simulink model "Virtual_Exhaust_Aftertreatment_Controller_PRT"  (R2016b)
settings: Solver=FixedStepAuto  StartTime=0.0  StopTime=inf  FixedStep=VirtExhATCtrlr.tiSimnTiStep_C  RelTol=1e-3  SampleTimeConstraint=STIndependent  EnableMultiTasking=on
undefined symbols (not defined in the file or in its folder): CAL, SOUIT, T3LIMCL_COEOM_MSK_SY, T3LimCL_stMskEOM1_C, T3LimCL_stMskEOM2_C, T3LimCL_stMskEOM3_C, VirtExhATCtrlr_numHrznSize_CA
libraries: simulink x4
(part 3 of 5)

== system Virtual_Exhaust_Aftertreatment_Controller_PRT/UCatCtrl/SCR_Prediction/Main/UCat NH3 Load Prediction ==
  ATS_tEstUCatAvrg : Inport
  ATS_mflEG : Inport  Port=2
  ATS_facEffUCatAge : Inport  Port=3
  ATS_mflNH3CurrEfc_mgps : Inport  Port=4
  ATS_mflNH3Cnv_mgps : Inport  Port=5
  ATS_stNH3LoadUCatRst : Inport  Port=6
  ATS_mflNH3MetAdapDes_mgps : Inport  Port=7
  ATS_mNH3LoadUCatRst : Inport  Port=8
  ATS_mNH3LoadUCatIni : Inport  Port=9
  Constant1 : Constant  Value=1000  SampleTime=-1
  Constant2 : Constant  Value=0  SampleTime=-1
  Constant6 : Constant  SampleTime=-1
  Constant_1 : Constant  Value=0.02  SampleTime=-1
  Discrete Integrator : Subsystem  mask(Discrete Integrator){}
      mask help:
      | X: Input value
      | Ki: Integral gain
      | Reset: Reset status
      | YReset: Output value during reset
      | Min: Minimum limit of output
      | Max: Maximum limit of output
      | dT : Discrete sample time [sec]
      | Y: Output value
      mask Display:
      | color('blue');
      | fprintf('Discrete\nIntegrator');
      | 
      | color('black');
      | port_label('input', 1, 'X');
      | port_label('input', 2, 'Ki');
      | port_label('input', 3, 'stReset');
      | port_label('input', 4, 'Y0(YReset)');
      | port_label('input', 5, 'Min');
      | port_label('input', 6, 'Max');
      | port_label('input', 7, 'dT');
      | port_label('output', 1, 'Y');
  Divide2 : Product  Inputs=*/
  GOTO_ATS_mflNH3OxiUCatUs_mgps : Subsystem  mask{SIG='ATS_mflNH3OxiUCatUs_mgps'}
      mask prompts: SIG "Log Signal Name"
      mask init: same as Virtual_Exhaust_Aftertreatment_Controller_PRT/UCatCtrl/SCR_Prediction/GOTO_ATS_etaEstNOxCnvUCat
      mask Display: fprintf(SIG);
  Interpolation Using Prelookup : Interpolation_n-D  NumberOfTableDimensions=1  TableSource=Input port  Table=|  ExtrapMethod=Clip  ValidIndexMayReachLast=on
      | [    0.2790    0.2970    0.3080    0.3220    0.3510    0.4240    0.5640    0.6550    0.8190    1.0000    1.0000    1.0000
      |     0.3260    0.3430    0.3540    0.3670    0.3960    0.4660    0.6010    0.6900    0.8440    1.0000    1.0000    1.0000
      |     0.3730    0.3890    0.4000    0.4130    0.4400    0.5080    0.6380    0.7230    0.8680    1.0000    1.0000    1.0000
      |     0.4320    0.4480    0.4580    0.4700    0.4960    0.5600    0.6830    0.7640    0.8970    1.0000    1.0000    1.0000
      |     0.4920    0.5070    0.5160    0.5270    0.5520    0.6120    0.7260    0.8020    0.9220    1.0000    1.0000    1.0000
      |     0.5510    0.5650    0.5730    0.5840    0.6070    0.6620    0.7680    0.8370    0.9410    1.0000    1.0000    1.0000
      |     0.6070    0.6200    0.6280    0.6380    0.6600    0.7130    0.8130    0.8750    0.9580    1.0000    1.0000    1.0000
      |     0.6580    0.6710    0.6790    0.6890    0.7110    0.7630    0.8600    0.9130    0.9730    1.0000    1.0000    1.0000
      |     0.7030    0.7170    0.7250    0.7360    0.7580    0.8130    0.9110    0.9540    0.9900    1.0000    1.0000    1.0000
      |     0.7620    0.7790    0.7900    0.8030    0.8300    0.8980    1.0000    1.0000    1.0000    1.0000    1.0000    1.0000
      |     0.7840    0.7980    0.8060    0.8160    0.8370    0.8910    0.9920    1.0000    1.0000    1.0000    1.0000    1.0000
      |     0.7800    0.8780    0.8820    0.8860    0.8950    0.9180    0.9620    1.0000    1.0000    1.0000    1.0000    1.0000
      | ]
      settings: InputPortMap=u0,u1,p2
  Lookup_n-D_2 : Lookup_n-D  NumberOfTableDimensions=1  BreakpointsForDimension1=[0;0.143;0.286;0.429;0.571;0.714;0.857;1]  Table=[0;0.143;0.286;0.429;0.571;0.714;0.857;1]  ExtrapMethod=Clip  UseLastTableValue=on  RndMeth=Simplest  InputSameDT=on
  Lookup_n-D_3 : Lookup_n-D  BreakpointsForDimension1=[189.96;209.96;229.96;249.96;299.96;349.96;399.96;449.96]  BreakpointsForDimension2=[0 120 200 300 580 700 1040 1500]  Table=[22 22 22 22 22 22 22 22;21.5 21.5 21.5 21.5 21.5 21.5 21.5 21.5;20.7000007629395 20.7000007629395 20.7000007629395 20.7000007629395 20.7000007629395 20.7000007629395 20.7000007629395 20.7000007629395;19.5 19.5 19.5 19.5 19.5 19.5 19.5 19.5;15.5 15.5 15.5 15.5 15.5 15.5 15.5 15.5;11.6999998092651 11.6999998092651 11.6999998092651 11.6999998092651 11.6999998092651 11.6999998092651 11.6999998092651 11.6999998092651;3.79999995231628 3.79999995231628 3.79999995231628 3.79999995231628 3.79999995231628 3.79999995231628 3.79999995231628 3.79999995231628;2.5 2.5 2.5 2.5 2.5 2.5 2.5 2.5]  ExtrapMethod=Clip  UseLastTableValue=on  RndMeth=Simplest  InputSameDT=on
  Lookup_n-D_4 : Lookup_n-D  BreakpointsForDimension1=[189.96;209.96;229.96;249.96;299.96;349.96;399.96;449.96]  BreakpointsForDimension2=[0 120 200 300 580 700 1040 1500]  Table=[29.5009994506836 29.5009994506836 29.5009994506836 29.5009994506836 29.5009994506836 29.5009994506836 29.5009994506836 29.5009994506836;28.2679996490479 28.2679996490479 28.2679996490479 28.2679996490479 28.2679996490479 28.2679996490479 28.2679996490479 28.2679996490479;26.0960006713867 26.0960006713867 26.0960006713867 26.0960006713867 26.0960006713867 26.0960006713867 26.0960006713867 26.0960006713867;22.8250007629395 22.8250007629395 22.8250007629395 22.8250007629395 22.8250007629395 22.8250007629395 22.8250007629395 22.8250007629395;18.5620002746582 18.5620002746582 18.5620002746582 18.5620002746582 18.5620002746582 18.5620002746582 18.5620002746582 18.5620002746582;13.4449996948242 13.4449996948242 13.4449996948242 13.4449996948242 13.4449996948242 13.4449996948242 13.4449996948242 13.4449996948242;4.65299987792969 4.65299987792969 4.65299987792969 4.65299987792969 4.65299987792969 4.65299987792969 4.65299987792969 4.65299987792969;2.49399995803833 2.49399995803833 2.49399995803833 2.49399995803833 2.49399995803833 2.49399995803833 2.49399995803833 2.49399995803833]  ExtrapMethod=Clip  UseLastTableValue=on  RndMeth=Simplest  InputSameDT=on
  Multiport Switch1 : MultiPortSwitch  DataPortOrder=Zero-based contiguous  Inputs=2
  Mux1 : Mux  Inputs=2
  NH3 Oxidation : Subsystem
  Prelookup : PreLookup  BreakpointsData=|  UseLastBreakpoint=on
      | [  0 1.0
      | ]
  Subtract : Sum  Inputs=+-
  Subtract1 : Sum  Inputs=+-
  ATS_mflNH3OxiUCatUs_mgps : Outport
  ATS_mEstNH3LdUCat : Outport  Port=2
  wires:
  ATS_tEstUCatAvrg/1 -> NH3 Oxidation/1(ATS_tEstUCatAvrg), Lookup_n-D_4/1, Lookup_n-D_3/1
  ATS_facEffUCatAge/1 -> NH3 Oxidation/4(ATS_facEffUCatAge), Lookup_n-D_2/1
  ATS_mflEG/1 -> NH3 Oxidation/2(ATS_mflEG), Lookup_n-D_4/2, Lookup_n-D_3/2
  ATS_mflNH3CurrEfc_mgps/1 -> Subtract/1
  Constant1/1 -> Divide2/2
  Divide2/1 -> Discrete Integrator/1(X)
  ATS_mflNH3Cnv_mgps/1 -> Subtract/2
  Discrete Integrator/1(Y) -> NH3 Oxidation/5(ATS_mEstNH3LdUCat), ATS_mEstNH3LdUCat/1
  Subtract/1 -> Subtract1/1
  Subtract1/1 -> Divide2/1
  NH3 Oxidation/1(ATS_mflNH3OxiUCatUs_mgps) -> GOTO_ATS_mflNH3OxiUCatUs_mgps/1(InXX), ATS_mflNH3OxiUCatUs_mgps/1, Subtract1/2
  Constant6/1 -> Discrete Integrator/2(Ki)
  Multiport Switch1/1 -> Discrete Integrator/4(Y0_YReset)
  ATS_stNH3LoadUCatRst/1 -> Multiport Switch1/1, Discrete Integrator/3(Reset)
  Constant_1/1 -> Discrete Integrator/7(dT)
  Interpolation Using Prelookup/1 -> Discrete Integrator/6(Max)
  Prelookup/1 -> Interpolation Using Prelookup/1
  Prelookup/2 -> Interpolation Using Prelookup/2
  Lookup_n-D_2/1 -> Prelookup/1
  Lookup_n-D_3/1 -> Mux1/1
  Lookup_n-D_4/1 -> Mux1/2
  Mux1/1 -> Interpolation Using Prelookup/3
  Constant2/1 -> Discrete Integrator/5(Min)
  ATS_mflNH3MetAdapDes_mgps/1 -> NH3 Oxidation/3(ATS_mflNH3MetAdapDes_mgps)
  ATS_mNH3LoadUCatIni/1 -> Multiport Switch1/2
  ATS_mNH3LoadUCatRst/1 -> Multiport Switch1/3

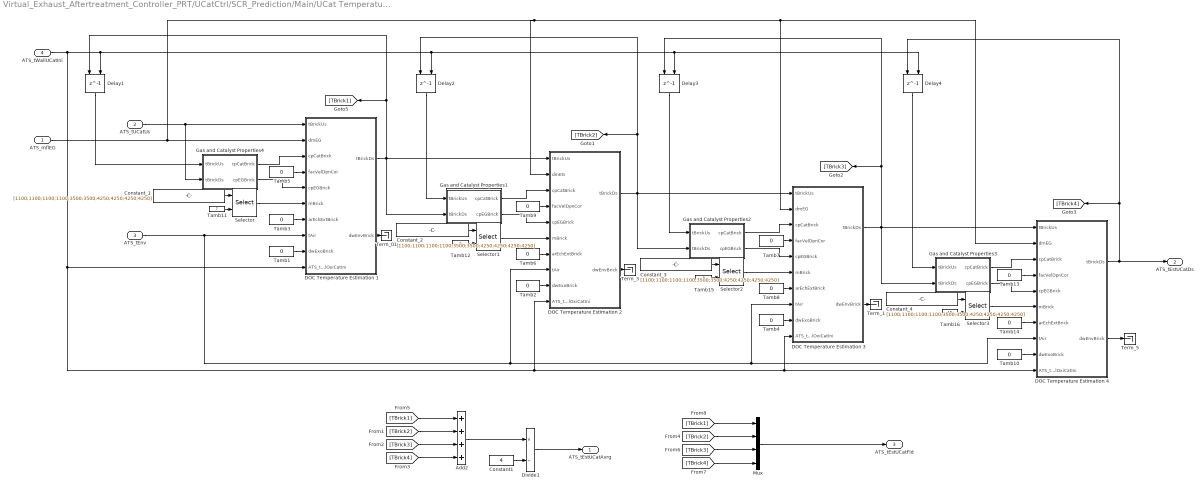
== system Virtual_Exhaust_Aftertreatment_Controller_PRT/UCatCtrl/SCR_Prediction/Main/UCat Temperature Prediction ==
  ATS_mflEG : Inport
  ATS_tUCatUs : Inport  Port=2
  ATS_tEnv : Inport  Port=3
  ATS_tWallUCatIni : Inport  Port=4
  Add2 : Sum  Inputs=++++
  Constant1 : Constant  Value=4  SampleTime=-1
  Constant_{1..4} (4 alike) : Constant  Description=THC DOC upstream  Value=[1100;1100;1100;1100;3500;3500;4250;4250;4250;4250]  SampleTime=-1
  DOC Temperature Estimation 1 : Subsystem  TreatAsAtomicUnit=on
  DOC Temperature Estimation 2 : Subsystem  TreatAsAtomicUnit=on
  DOC Temperature Estimation 3 : Subsystem  TreatAsAtomicUnit=on
  DOC Temperature Estimation 4 : Subsystem  TreatAsAtomicUnit=on
  Delay{1..4} (4 alike) : Delay  DelayLength=1  InitialConditionSource=Input port  InitialCondition=0
      settings: InputPortMap=u0,p4
  Divide1 : Product  Inputs=*/
  Gas and Catalyst Properties1 : Subsystem  TreatAsAtomicUnit=on
  Gas and Catalyst Properties2 : Subsystem  TreatAsAtomicUnit=on
  Gas and Catalyst Properties3 : Subsystem  TreatAsAtomicUnit=on
  Gas and Catalyst Properties4 : Subsystem  TreatAsAtomicUnit=on
  Mux : Mux
  Selector{,1..3} (4 alike) : Selector  InputPortWidth=10  IndexOptions=Index vector (port)  Indices=[1 3]  OutputSizes=1
  Tamb{1..10,13..14} (12 alike) : Constant  Value=0  SampleTime=-1
  Tamb11 : Constant  Value=7  SampleTime=-1
  Tamb12 : Constant  Value=8  SampleTime=-1
  Tamb15 : Constant  Value=9  SampleTime=-1
  Tamb16 : Constant  Value=10  SampleTime=-1
  Term_01 : Terminator
  Term_1 : Terminator
  Term_3 : Terminator
  Term_5 : Terminator
  ATS_tEstUCatAvrg : Outport
  ATS_tEstUCatDs : Outport  Port=2
  ATS_tEstUCatFld : Outport  Port=3
  wires:
  ATS_tUCatUs/1 -> Gas and Catalyst Properties4/2(tBrickDs), DOC Temperature Estimation 1/1(tBrickUs)
  Gas and Catalyst Properties4/2(cpEGBrick) -> DOC Temperature Estimation 1/5(cpEGBrick)
  Gas and Catalyst Properties4/1(cpCatBrick) -> DOC Temperature Estimation 1/3(cpCatBrick)
  Tamb5/1 -> DOC Temperature Estimation 1/4(facVelDpnCor)
  Tamb3/1 -> DOC Temperature Estimation 1/7(arEchExtBrick)
  DOC Temperature Estimation 1/2(dwEnvBrick) -> Term_01/1
  DOC Temperature Estimation 1/1(tBrickDs) -> Gas and Catalyst Properties1/2(tBrickDs), DOC Temperature Estimation 2/1(tBrickUs), [TBrick1], Delay1/1
  Delay1/1 -> Gas and Catalyst Properties4/1(tBrickUs)
  Gas and Catalyst Properties3/2(cpEGBrick) -> DOC Temperature Estimation 4/5(cpEGBrick)
  Gas and Catalyst Properties3/1(cpCatBrick) -> DOC Temperature Estimation 4/3(cpCatBrick)
  Delay4/1 -> Gas and Catalyst Properties3/1(tBrickUs)
  Gas and Catalyst Properties2/2(cpEGBrick) -> DOC Temperature Estimation 3/5(cpEGBrick)
  Gas and Catalyst Properties2/1(cpCatBrick) -> DOC Temperature Estimation 3/3(cpCatBrick)
  Delay3/1 -> Gas and Catalyst Properties2/1(tBrickUs)
  Gas and Catalyst Properties1/2(cpEGBrick) -> DOC Temperature Estimation 2/5(cpEGBrick)
  Gas and Catalyst Properties1/1(cpCatBrick) -> DOC Temperature Estimation 2/3(cpCatBrick)
  Delay2/1 -> Gas and Catalyst Properties1/1(tBrickUs)
  DOC Temperature Estimation 2/1(tBrickDs) -> Gas and Catalyst Properties2/2(tBrickDs), DOC Temperature Estimation 3/1(tBrickUs), [TBrick2], Delay2/1
  DOC Temperature Estimation 4/2(dwEnvBrick) -> Term_5/1
  DOC Temperature Estimation 4/1(tBrickDs) -> Delay4/1, [TBrick4], ATS_tEstUCatDs/1
  ATS_tEnv/1 -> DOC Temperature Estimation 1/8(tAir), DOC Temperature Estimation 2/8(tAir), DOC Temperature Estimation 4/8(tAir), DOC Temperature Estimation 3/8(tAir)
  Tamb14/1 -> DOC Temperature Estimation 4/7(arEchExtBrick)
  DOC Temperature Estimation 3/2(dwEnvBrick) -> Term_1/1
  Tamb13/1 -> DOC Temperature Estimation 4/4(facVelDpnCor)
  DOC Temperature Estimation 3/1(tBrickDs) -> Gas and Catalyst Properties3/2(tBrickDs), DOC Temperature Estimation 4/1(tBrickUs), [TBrick3], Delay3/1
  Tamb8/1 -> DOC Temperature Estimation 3/7(arEchExtBrick)
  Tamb7/1 -> DOC Temperature Estimation 3/4(facVelDpnCor)
  Tamb9/1 -> DOC Temperature Estimation 2/4(facVelDpnCor)
  Tamb6/1 -> DOC Temperature Estimation 2/7(arEchExtBrick)
  DOC Temperature Estimation 2/2(dwEnvBrick) -> Term_3/1
  Constant1/1 -> Divide1/2
  Add2/1 -> Divide1/1
  [TBrick4] -> Add2/4
  [TBrick3] -> Add2/3
  [TBrick2] -> Add2/2
  [TBrick1] -> Add2/1
  [TBrick4] -> Mux/4
  [TBrick3] -> Mux/3
  [TBrick2] -> Mux/2
  [TBrick1] -> Mux/1
  Mux/1 -> ATS_tEstUCatFld/1
  Divide1/1 -> ATS_tEstUCatAvrg/1
  ATS_tWallUCatIni/1 -> DOC Temperature Estimation 2/10(ATS_tWallOxiCatIni), DOC Temperature Estimation 4/10(ATS_tWallOxiCatIni), DOC Temperature Estimation 3/10(ATS_tWallOxiCatIni), DOC Temperature Estimation 1/10(ATS_tWallOxiCatIni), Delay4/2, Delay3/2, Delay2/2, Delay1/2
  ATS_mflEG/1 -> DOC Temperature Estimation 2/2(dmEG), DOC Temperature Estimation 4/2(dmEG), DOC Temperature Estimation 3/2(dmEG), DOC Temperature Estimation 1/2(dmEG)
  Selector1/1 -> DOC Temperature Estimation 2/6(mBrick)
  Selector2/1 -> DOC Temperature Estimation 3/6(mBrick)
  Selector3/1 -> DOC Temperature Estimation 4/6(mBrick)
  Tamb1/1 -> DOC Temperature Estimation 1/9(dwExoBrick)
  Tamb2/1 -> DOC Temperature Estimation 2/9(dwExoBrick)
  Tamb4/1 -> DOC Temperature Estimation 3/9(dwExoBrick)
  Tamb10/1 -> DOC Temperature Estimation 4/9(dwExoBrick)
  Selector/1 -> DOC Temperature Estimation 1/6(mBrick)
  Constant_1/1 -> Selector/1
  Tamb11/1 -> Selector/2
  Constant_2/1 -> Selector1/1
  Tamb12/1 -> Selector1/2
  Constant_3/1 -> Selector2/1
  Tamb15/1 -> Selector2/2
  Constant_4/1 -> Selector3/1
  Tamb16/1 -> Selector3/2

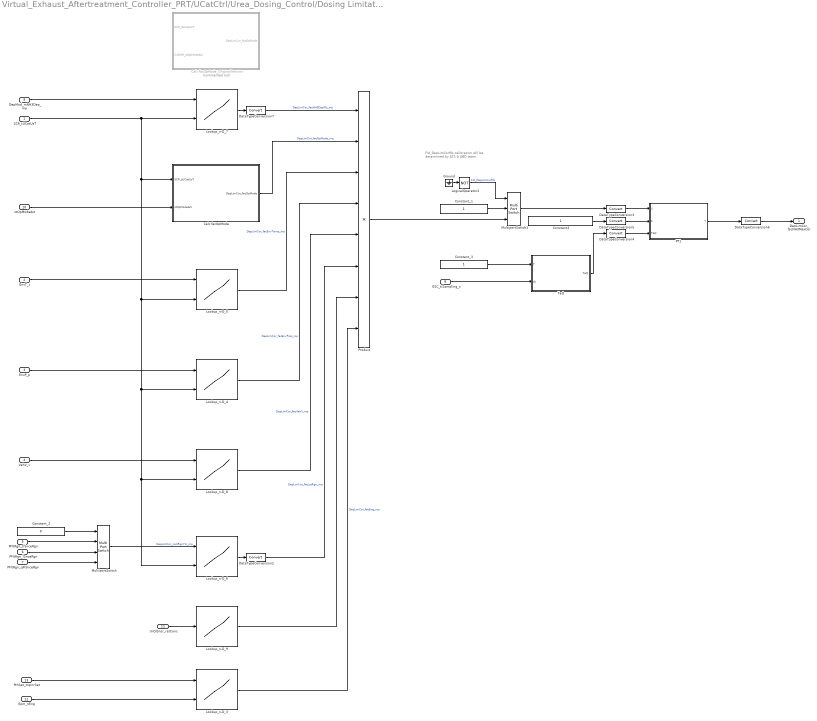
== system Virtual_Exhaust_Aftertreatment_Controller_PRT/UCatCtrl/Urea_Dosing_Control/Dosing Limitation/DepLimCor ==
  note: FId_DepLimCorRls calibration will be
      | determined by ATS & OBD team.
  SCR_tUCatUsT : Inport
  EnvT_t : Inport  Port=2
  EnvP_p : Inport  Port=3
  VehV_v : Inport  Port=4
  PFltRgn_tiSnceRgn : Inport  Port=5
  PFltRgn_lSnceRgn : Inport  Port=6
  PFltRgn_qFlSnceRgn : Inport  Port=7
  ESC_tiSampling_s : Inport  Port=8
  DepMod_mNH3Dep_mp : Inport  Port=9
  stOpModeAct : Inport  Port=10
  UrQlSnsr_ratConc : Inport  Port=11
  Epm_nEng : Inport  Port=12
  PthSet_trqInrSet : Inport  Port=13
  " Calc facOpMode" : Subsystem
  " Calc facOpMode_OriginalVersion" : Subsystem  Commented=on
  Constant3 : Constant  OutDataTypeStr=Inherit: Inherit via back propagation
  Constant_1 : Constant  SampleTime=-1
  Constant_2 : Constant  Value=0  SampleTime=-1
  Constant_3 : Constant  SampleTime=-1
  DataTypeConversion{2..7} (6 alike) : DataTypeConversion  RndMeth=Simplest  SaturateOnIntegerOverflow=on
  Ground : Ground
  LogicalOperator2 : Logic  Operator=NOT  AllPortsSameDT=off  OutDataTypeStr=boolean
  Lookup_n-D_3 : Lookup_n-D  BreakpointsForDimension1=[0;3;200;300;400;500;600;700;800;900;1000;1100;1200;1300;1400;1500;1600;1700;1800;1900;2000;2100;2200;2300]  BreakpointsForDimension2=[600 700 750 800 850 900 950 1000 1050 1100 1150 1200 1250 1300 1350 1400 1450 1500 1550 1600 1650 1700 1750 1800]  Table=[0 0 0 0 0 0 0 0 0 0 0 0 0 0 0 0 0 0 0 0 0 0 0 0;1 1 1 1 1 1 1 1 1 1 1 1 1 1 1 1 1 1 1 1 1 1 1 1;1 1 1 1 1 1 1 1 1 1 1 1 1 1 1 1 1 1 1 1 1 1 1 1;1 1 1 1 1 1 1 1 1 1 1 1 1 1 1 1 1 1 1 1 1 1 1 1;1 1 1 1 1 1 1 1 1 1 1 1 1 1 1 1 1 1 1 1 1 1 1 1;1 1 1 1 1 1 1 1 1 1 1 1 1 1 1 1 1 1 1 1 1 1 1 1;1 1 1 1 1 1 1 1 1 1 1 1 1 1 1 1 1 1 1 1 1 1 1 1;1 1 1 1 1 1 1 1 1 1 1 1 1 1 1 1 1 1 1 1 1 1 1 1;1 1 1 1 1 1 1 1 1 1 1 1 1 1 1 1 1 1 1 1 1 1 1 1;1 1 1 1 1 1 1 1 1 1 1 1 1 1 1 1 1 1 1 1 1 1 1 1;1 1 1 1 1 1 1 1 1 1 1 1 1 1 1 1 1 1 1 1 1 1 1 1;1 1 1 1 1 1 1 1 1 1 1 1 1 1 1 1 1 1 1 1 1 1 1 1;1 1 1 1 1 1 1 1 1 1 1 1 1 1 1 1 1 1 1 1 1 1 1 1;1 1 1 1 1 1 1 1 1 1 1 1 1 1 1 1 1 1 1 1 1 1 1 1;1 1 1 1 1 1 1 1 1 1 1 1 1 1 1 1 1 1 1 1 1 1 1 1;1 1 1 1 1 1 1 1 1 1 1 1 1 1 1 1 1 1 1 1 1 1 1 1;1 1 1 1 1 1 1 1 1 1 1 1 1 1 1 1 1 1 1 1 1 1 1 1;1 1 1 1 1 1 1 1 1 1 1 1 1 1 1 1 1 1 1 1 1 1 1 1;1 1 1 1 1 1 1 1 1 1 1 1 1 1 1 1 1 1 1 1 1 1 1 1;1 1 1 1 1 1 1 1 1 1 1 1 1 1 1 1 1 1 1 1 1 1 1 1;1 1 1 1 1 1 1 1 1 1 1 1 1 1 1 1 1 1 1 1 1 1 1 1;1 1 1 1 1 1 1 1 1 1 1 1 1 1 1 1 1 1 1 1 1 1 1 1;1 1 1 1 1 1 1 1 1 1 1 1 1 1 1 1 1 1 1 1 1 1 1 1;1 1 1 1 1 1 1 1 1 1 1 1 1 1 1 1 1 1 1 1 1 1 1 1]  ExtrapMethod=Clip  UseLastTableValue=on  RndMeth=Simplest  InputSameDT=on
  Lookup_n-D_4 : Lookup_n-D  BreakpointsForDimension1=[100;750;800;840;845;1000;1040;1080]  BreakpointsForDimension2=[159.96 189.96 229.96 249.96 299.96 349.96 399.96 599.96]  Table=[0 0 0 0 0 0 0 0;0.4 0.4 0.4 0.4 0.4 0.4 0.4 0.4;0.5 0.5 0.5 0.5 0.5 0.5 0.5 0.5;0.75 0.75 0.75 0.75 0.75 0.75 0.75 0.75;1 1 1 1 1 1 1 1;1 1 1 1 1 1 1 1;1 1 1 1 1 1 1 1;1 1 1 1 1 1 1 1]  ExtrapMethod=Clip  UseLastTableValue=on  RndMeth=Simplest  InputSameDT=on
  Lookup_n-D_5 : Lookup_n-D  BreakpointsForDimension1=[-11.04;-8.04000000000001;-7.04000000000001;-0.0400000000000091;4.95999999999999;14.96;34.96;37.96]  BreakpointsForDimension2=[159.96 189.96 219.96 249.96 299.96 349.96 399.96 599.96]  Table=[1 1 1 1 1 1 1 1;1 1 1 1 1 1 1 1;1 1 1 1 1 1 1 1;1 1 1 1 1 1 1 1;1 1 1 1 1 1 1 1;1 1 1 1 1 1 1 1;1 1 1 1 1 1 1 1;1 1 1 1 1 1 1 1]  ExtrapMethod=Clip  UseLastTableValue=on  RndMeth=Simplest  InputSameDT=on
  Lookup_n-D_6 : Lookup_n-D  BreakpointsForDimension1=[0;2000;6000;10000;14000;18000;20000;60000]  BreakpointsForDimension2=[159.960006713867 190 229.960006713867 249.960006713867 299.959991455078 349.959991455078 399.959991455078 599.960021972656]  Table=[0 1 1 1 1 1 1 1;0 1 1 1 1 1 1 1;0 1 1 1 1 1 1 1;0 1 1 1 1 1 1 1;0 1 1 1 1 1 1 1;0 1 1 1 1 1 1 1;0 1 1 1 1 1 1 1;0 0.899999976158142 0.899999976158142 0.899999976158142 1 1 1 1]  ExtrapMethod=Clip  UseLastTableValue=on  RndMeth=Simplest  InputSameDT=on
  Lookup_n-D_7 : Lookup_n-D  BreakpointsForDimension1=[0;2;5;10;15;20;25;30]  BreakpointsForDimension2=[159.960006713867 190 229.960006713867 249.960006713867 299.959991455078 349.959991455078 399.959991455078 599.960021972656]  Table=[0 1 1 1 1 1 1 1;0 1 1 1 1 1 1 1;0 1 1 1 1 1 1 1;0 1 1 1 1 1 1 1;0 1 1 1 1 1 1 1;0 0.75 1 1 1 1 1 1;0 0.600000023841858 1 1 1 1 1 1;0 0.5 1 1 1 1 1 1]  ExtrapMethod=Clip  UseLastTableValue=on  RndMeth=Simplest  InputSameDT=on
  Lookup_n-D_8 : Lookup_n-D  BreakpointsForDimension1=[0;10;20;40;60;80;100;120]  BreakpointsForDimension2=[159.96 199.96 229.96 249.96 299.96 349.96 399.96 599.96]  Table=[1 1 1 1 1 1 1 1;1 1 1 1 1 1 1 1;1 1 1 1 1 1 1 1;1 1 1 1 1 1 1 1;1 1 1 1 1 1 1 1;1 1 1 1 1 1 1 1;1 1 1 1 1 1 1 1;1 1 1 1 1 1 1 1]  ExtrapMethod=Clip  UseLastTableValue=on  RndMeth=Simplest  InputSameDT=on
  Lookup_n-D_9 : Lookup_n-D  NumberOfTableDimensions=1  BreakpointsForDimension1=[18;19;20;22.5;25;30.5;32.5]  BreakpointsForDimension2=[159.96 449.96]  Table=[0.8;1.22;1.2;1.05;1.02;1;1]  ExtrapMethod=Clip  UseLastTableValue=on  RndMeth=Simplest  InputSameDT=on
  MultiportSwitch : MultiPortSwitch  DataPortOrder=Zero-based contiguous
  MultiportSwitch1 : MultiPortSwitch  DataPortOrder=Zero-based contiguous  Inputs=2
  PT1 : Subsystem
  Product : Product  Inputs=8  OutDataTypeStr=Inherit: Inherit via back propagation  RndMeth=Simplest  SaturateOnIntegerOverflow=on
  TeQ : Subsystem
  DepLimCor_facNH3MaxCor : Outport
  wires:
  EnvT_t/1 -> Lookup_n-D_5/1
  Lookup_n-D_5/1 -> Product/3  "DepLimCor_facEnvTemp_mp"
  EnvP_p/1 -> Lookup_n-D_4/1
  Lookup_n-D_4/1 -> Product/4  "DepLimCor_facEnvPres_mp"
  VehV_v/1 -> Lookup_n-D_8/1
  Lookup_n-D_8/1 -> Product/5  "DepLimCor_facVehV_mp"
  Constant_2/1 -> MultiportSwitch/1
  DataTypeConversion2/1 -> Product/6  "DepLimCor_facLstRgn_mp"
  Product/1 -> MultiportSwitch1/3
  Constant_1/1 -> MultiportSwitch1/2
  Lookup_n-D_6/1 -> DataTypeConversion2/1
  MultiportSwitch1/1 -> DataTypeConversion3/1
  Constant3/1 -> DataTypeConversion5/1
  DataTypeConversion3/1 -> PT1/1(X)
  DataTypeConversion4/1 -> PT1/3(TeQ)
  DataTypeConversion5/1 -> PT1/2(K)
  Constant_3/1 -> TeQ/1(T)
  TeQ/1(TeQ) -> DataTypeConversion4/1
  ESC_tiSampling_s/1 -> TeQ/2(dt)
  DataTypeConversion6/1 -> DepLimCor_facNH3MaxCor/1
  DepMod_mNH3Dep_mp/1 -> Lookup_n-D_7/1
  Lookup_n-D_7/1 -> DataTypeConversion7/1
  DataTypeConversion7/1 -> Product/1  "DepLimCor_facNH3DepMs_mp"
  stOpModeAct/1 -> " Calc facOpMode"/2(stOpModeAct)
  " Calc facOpMode"/1(DepLimCor_facOpMode) -> Product/2  "DepLimCor_facOpMode_mp"
  SCR_tUCatUsT/1 -> Lookup_n-D_7/2, " Calc facOpMode"/1(SCR_tUCatUsT), Lookup_n-D_5/2, Lookup_n-D_4/2, Lookup_n-D_6/2, Lookup_n-D_8/2
  PFltRgn_tiSnceRgn/1 -> MultiportSwitch/2
  PFltRgn_lSnceRgn/1 -> MultiportSwitch/3
  PFltRgn_qFlSnceRgn/1 -> MultiportSwitch/4
  MultiportSwitch/1 -> Lookup_n-D_6/1  "DepLimCor_xLstRgnYIn_mp"
  UrQlSnsr_ratConc/1 -> Lookup_n-D_9/1
  PT1/1(Y) -> DataTypeConversion6/1
  Lookup_n-D_9/1 -> Product/7
  Epm_nEng/1 -> Lookup_n-D_3/2
  PthSet_trqInrSet/1 -> Lookup_n-D_3/1
  Lookup_n-D_3/1 -> Product/8  "DepLimCor_facEng_mp"
  Ground/1 -> LogicalOperator2/1
  LogicalOperator2/1 -> MultiportSwitch1/1  "FId_DepLimCorRls"

== system Virtual_Exhaust_Aftertreatment_Controller_PRT/UCatCtrl/Urea_Dosing_Control/Dosing Limitation/GOTO_DepLimCor_facNH3MaxCor ==
  InXX : Inport
  GainXX : Subsystem
  tag scope: DepLimCor_facNH3MaxCor=global
  wires:
  GainXX/1(Out) -> [DepLimCor_facNH3MaxCor]  "DepLimCor_facNH3MaxCor"
  InXX/1 -> GainXX/1(In)

== system Virtual_Exhaust_Aftertreatment_Controller_PRT/UCatCtrl/Urea_Dosing_Control/Dosing Limitation/GOTO_SCRLdG_dmNH3Max ==
  InXX : Inport
  GainXX : Subsystem
  tag scope: SCRLdG_dmNH3Max=global
  wires:
  InXX/1 -> GainXX/1(In)
  GainXX/1(Out) -> [SCRLdG_dmNH3Max]  "SCRLdG_dmNH3Max"

== system Virtual_Exhaust_Aftertreatment_Controller_PRT/UCatCtrl/Urea_Dosing_Control/EvpMod/EvpMod_HtFlwPostReac ==
  note: (NH_2)_2CO + H_2O \rightarrow 2NH_3 + CO_2
  note: Molar mass of water
  note: Molar mass of urea
  note: Molar mass of NH3
  note: Molar mass of urea
  note: Molar mass of CO2
  note: Molar mass of urea
  dmUrea : Inport
  dmWtVapo : Inport  Port=2
  cpWtPostReac : Inport  Port=3
  tUCatUsT : Inport  Port=4
  cpNH3 : Inport  Port=5
  cpCO2 : Inport  Port=6
  Constant_1 : Constant  Value=60
  Constant_10 : Constant  Value=60
  Constant_2 : Constant  Value=18
  Constant_3 : Constant  Value=1475.17004394531  SampleTime=-1
  Constant_4 : Constant  Value=60
  Constant_5 : Constant  Value=2
  Constant_6 : Constant  Value=133  SampleTime=-1
  Constant_7 : Constant  Value=17
  Constant_9 : Constant  Value=44
  Divide : Product  Inputs=*/  RndMeth=Simplest  SaturateOnIntegerOverflow=on
  Divide1 : Product  Inputs=*/  RndMeth=Simplest  SaturateOnIntegerOverflow=on
  Divide2 : Product  Inputs=*/  RndMeth=Simplest  SaturateOnIntegerOverflow=on
  Product{1..9,11..12} (11 alike) : Product
  Subtract : Sum  Inputs=+-  RndMeth=Simplest  SaturateOnIntegerOverflow=on
  Subtract1 : Sum  Inputs=+-  RndMeth=Simplest  SaturateOnIntegerOverflow=on
  dwUreaReac : Outport
  dwWtPostReac : Outport  Port=2
  dwNH3 : Outport  Port=3
  dwCO2 : Outport  Port=4
  wires:
  Constant_3/1 -> Product11/2
  dmUrea/1 -> Product11/1, Product12/1, Product7/1, Product4/1
  Product11/1 -> dwUreaReac/1  "EvpMod_dwUreaReac_mp"
  Subtract1/1 -> Product2/1
  tUCatUsT/1 -> Subtract/1
  Constant_6/1 -> Subtract/2
  Subtract/1 -> Product1/2, Product8/1, Product6/1
  Product1/1 -> Product2/2
  Product2/1 -> dwWtPostReac/1  "EvpMod_dwWtPostReac_mp"
  dmWtVapo/1 -> Subtract1/1
  Product12/1 -> Subtract1/2
  Constant_2/1 -> Divide/1
  Constant_4/1 -> Divide/2
  Divide/1 -> Product12/2
  cpWtPostReac/1 -> Product1/1
  Divide1/1 -> Product4/2
  Constant_7/1 -> Product3/1
  Product5/1 -> dwNH3/1  "EvpMod_dwNH3_mp"
  Product6/1 -> Product5/2
  Product4/1 -> Product5/1
  Product3/1 -> Divide1/1
  Constant_5/1 -> Product3/2
  Constant_1/1 -> Divide1/2
  cpNH3/1 -> Product6/2
  Constant_10/1 -> Divide2/2
  Product7/1 -> Product9/1
  Product8/1 -> Product9/2
  Product9/1 -> dwCO2/1  "EvpMod_dwCO2_mp"
  Divide2/1 -> Product7/2
  Constant_9/1 -> Divide2/1
  cpCO2/1 -> Product8/2

== system Virtual_Exhaust_Aftertreatment_Controller_PRT/UCatCtrl/Urea_Dosing_Control/EvpMod/EvpMod_HtFlwPreReac ==
  dmRdcAgCnv : Inport
  cpRdcAg : Inport  Port=2
  tUTnkT : Inport  Port=3
  dmWtVapo : Inport  Port=4
  dmUrea : Inport  Port=5
  cpUrea : Inport  Port=6
  cpWtPreReac : Inport  Port=7
  Constant_1 : Constant  Value=2257  SampleTime=-1
  Constant_2 : Constant  Value=133  SampleTime=-1
  Constant_3 : Constant  Value=100  SampleTime=-1
  Constant_4 : Constant  Value=100  SampleTime=-1
  Product{1..7} (7 alike) : Product
  Subtract : Sum  Inputs=+-  RndMeth=Simplest  SaturateOnIntegerOverflow=on
  Subtract1 : Sum  Inputs=+-  RndMeth=Simplest  SaturateOnIntegerOverflow=on
  dwRdcAg : Outport
  dwPhChngWt : Outport  Port=2
  dwUrea : Outport  Port=3
  dwWtPreReac : Outport  Port=4
  wires:
  dmRdcAgCnv/1 -> Product1/1
  Constant_4/1 -> Subtract/1
  tUTnkT/1 -> Subtract/2
  Subtract/1 -> Product7/2
  Product7/1 -> Product1/2
  Product1/1 -> dwRdcAg/1  "EvpMod_dwRdcAg_mp"
  cpRdcAg/1 -> Product7/1
  Constant_1/1 -> Product2/2
  Product2/1 -> dwPhChngWt/1  "EvpMod_dwPhChngWt_mp"
  dmWtVapo/1 -> Product6/1, Product2/1
  dmUrea/1 -> Product4/1
  Constant_2/1 -> Subtract1/1
  Constant_3/1 -> Subtract1/2
  Subtract1/1 -> Product5/1, Product3/2
  Product3/1 -> Product4/2
  Product4/1 -> dwUrea/1  "EvpMod_dwUrea_mp"
  cpUrea/1 -> Product3/1
  Product5/1 -> Product6/2
  Product6/1 -> dwWtPreReac/1  "EvpMod_dwWtPreReac_mp"
  cpWtPreReac/1 -> Product5/2

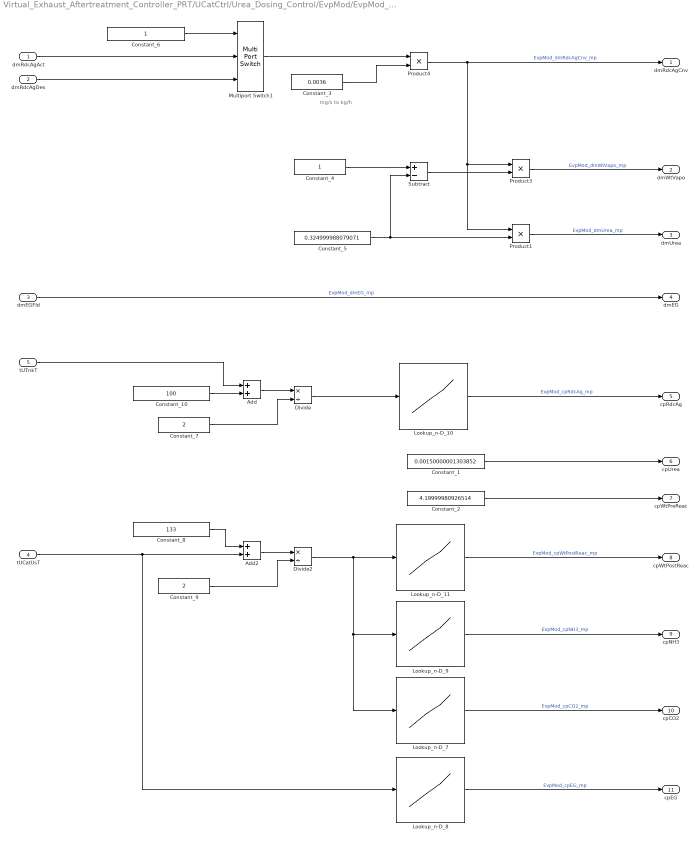
== system Virtual_Exhaust_Aftertreatment_Controller_PRT/UCatCtrl/Urea_Dosing_Control/EvpMod/EvpMod_InSigHdl ==
  note: mg/s to kg/h
  dmRdcAgAct : Inport
  dmRdcAgDes : Inport  Port=2
  dmEGFId : Inport  Port=3
  tUCatUsT : Inport  Port=4
  tUTnkT : Inport  Port=5
  Add : Sum  RndMeth=Simplest  SaturateOnIntegerOverflow=on
  Add2 : Sum  RndMeth=Simplest  SaturateOnIntegerOverflow=on
  Constant_1 : Constant  Value=0.00150000001303852  SampleTime=-1
  Constant_10 : Constant  Value=100  SampleTime=-1
  Constant_2 : Constant  Value=4.19999980926514  SampleTime=-1
  Constant_3 : Constant  Value=0.0036
  Constant_4 : Constant
  Constant_5 : Constant  Value=0.324999988079071  SampleTime=-1
  Constant_6 : Constant  SampleTime=-1
  Constant_7 : Constant  Value=2
  Constant_8 : Constant  Value=133  SampleTime=-1
  Constant_9 : Constant  Value=2
  Divide : Product  Inputs=*/  RndMeth=Simplest  SaturateOnIntegerOverflow=on
  Divide2 : Product  Inputs=*/  RndMeth=Simplest  SaturateOnIntegerOverflow=on
  Lookup_n-D_10 : Lookup_n-D  NumberOfTableDimensions=1  BreakpointsForDimension1=[0;25.0400009155273;45.0400009155273;65.0199966430664;65.0299987792969;65.0400009155273]  BreakpointsForDimension2=[159.96 449.96]  Table=[0.111000001430512;0.111000001430512;0.112999998033047;0.115000002086163;0.115000002086163;0.115000002086163]  ExtrapMethod=Clip  UseLastTableValue=on  RndMeth=Simplest  InputSameDT=on
  Lookup_n-D_11 : Lookup_n-D  NumberOfTableDimensions=1  BreakpointsForDimension1=[25;220;260;300;340;360]  BreakpointsForDimension2=[159.96 449.96]  Table=[4.18160009384155;4.61460018157959;4.98559999465942;5.75040006637573;8.20800018310547;15.003999710083]  ExtrapMethod=Clip  UseLastTableValue=on  RndMeth=Simplest  InputSameDT=on
  Lookup_n-D_7 : Lookup_n-D  NumberOfTableDimensions=1  BreakpointsForDimension1=[77;177;277;377;477;777]  BreakpointsForDimension2=[159.96 449.96]  Table=[0.894999980926514;0.977999985218048;1.0460000038147;1.10199999809265;1.14800000190735;1.24699997901917]  ExtrapMethod=Clip  UseLastTableValue=on  RndMeth=Simplest  InputSameDT=on
  Lookup_n-D_8 : Lookup_n-D  NumberOfTableDimensions=1  BreakpointsForDimension1=[77;127;227;327;527;727]  BreakpointsForDimension2=[159.96 449.96]  Table=[1.00899994373322;1.02100002765656;1.02999997138977;1.05099999904633;1.09899997711182;1.14100003242493]  ExtrapMethod=Clip  UseLastTableValue=on  RndMeth=Simplest  InputSameDT=on
  Lookup_n-D_9 : Lookup_n-D  NumberOfTableDimensions=1  BreakpointsForDimension1=[27;127;227;327;427;727]  BreakpointsForDimension2=[159.96 449.96]  Table=[2.09999990463257;2.27940011024475;2.47239995002747;2.66240000724792;2.84409999847412;3.32349991798401]  ExtrapMethod=Clip  UseLastTableValue=on  RndMeth=Simplest  InputSameDT=on
  Multiport Switch1 : MultiPortSwitch  DataPortOrder=Zero-based contiguous  Inputs=2
  Product1 : Product
  Product3 : Product
  Product4 : Product
  Subtract : Sum  Inputs=+-  RndMeth=Simplest  SaturateOnIntegerOverflow=on
  dmRdcAgCnv : Outport
  dmWtVapo : Outport  Port=2
  dmUrea : Outport  Port=3
  dmEG : Outport  Port=4
  cpRdcAg : Outport  Port=5
  cpUrea : Outport  Port=6
  cpWtPreReac : Outport  Port=7
  cpWtPostReac : Outport  Port=8
  cpNH3 : Outport  Port=9
  cpCO2 : Outport  Port=10
  cpEG : Outport  Port=11
  wires:
  Constant_4/1 -> Subtract/1
  Constant_5/1 -> Product1/2, Subtract/2
  Subtract/1 -> Product3/2
  Product3/1 -> dmWtVapo/1  "EvpMod_dmWtVapo_mp"
  Product1/1 -> dmUrea/1  "EvpMod_dmUrea_mp"
  Constant_3/1 -> Product4/2
  Product4/1 -> dmRdcAgCnv/1, Product1/1, Product3/1  "EvpMod_dmRdcAgCnv_mp"
  dmEGFId/1 -> dmEG/1  "EvpMod_dmEG_mp"
  Lookup_n-D_10/1 -> cpRdcAg/1  "EvpMod_cpRdcAg_mp"
  Lookup_n-D_9/1 -> cpNH3/1  "EvpMod_cpNH3_mp"
  Lookup_n-D_7/1 -> cpCO2/1  "EvpMod_cpCO2_mp"
  Lookup_n-D_8/1 -> cpEG/1  "EvpMod_cpEG_mp"
  tUTnkT/1 -> Add/1
  Constant_10/1 -> Add/2
  Add/1 -> Divide/1
  Constant_7/1 -> Divide/2
  Divide/1 -> Lookup_n-D_10/1
  Constant_8/1 -> Add2/1
  Add2/1 -> Divide2/1
  Constant_9/1 -> Divide2/2
  Divide2/1 -> Lookup_n-D_11/1, Lookup_n-D_9/1, Lookup_n-D_7/1
  tUCatUsT/1 -> Lookup_n-D_8/1, Add2/2
  Lookup_n-D_11/1 -> cpWtPostReac/1  "EvpMod_cpWtPostReac_mp"
  Constant_6/1 -> Multiport Switch1/1
  Multiport Switch1/1 -> Product4/1
  dmRdcAgDes/1 -> Multiport Switch1/3
  dmRdcAgAct/1 -> Multiport Switch1/2
  Constant_1/1 -> cpUrea/1
  Constant_2/1 -> cpWtPreReac/1

== system Virtual_Exhaust_Aftertreatment_Controller_PRT/UCatCtrl/Urea_Dosing_Control/EvpMod/EvpMod_UCatUsTEst ==
  note: Function initialization
  dwRdcAg : Inport
  dwPhChngWt : Inport  Port=2
  dwUrea : Inport  Port=3
  dwWtPreReac : Inport  Port=4
  dwUreaReac : Inport  Port=5
  dwWtPostReac : Inport  Port=6
  dwNH3 : Inport  Port=7
  dwCO2 : Inport  Port=8
  tUCatUsT : Inport  Port=9
  dmEG : Inport  Port=10
  cpEG : Inport  Port=11
  tiSampling : Inport  Port=12
  Add2 : Sum  Inputs=8
  Constant_1 : Constant  SampleTime=-1
  Constant_18 : Constant  Value=false  OutDataTypeStr=boolean
  Constant_2 : Constant  Value=800  SampleTime=-1
  Constant_3 : Constant  Value=0  SampleTime=-1
  Constant_4 : Constant
  Constant_5 : Constant  Value=150  SampleTime=-1
  Constant_6 : Constant  Value=5  SampleTime=-1
  Divide : Product  Inputs=*/  RndMeth=Simplest  SaturateOnIntegerOverflow=on
  Ground : Ground
  LogicalOperator : Logic  Operator=NOT  AllPortsSameDT=off  OutDataTypeStr=boolean
  LogicalOperator1 : Logic  Operator=OR  AllPortsSameDT=off  OutDataTypeStr=boolean
  LogicalOperator2 : Logic  Operator=NOT  AllPortsSameDT=off  OutDataTypeStr=boolean
  MinMax : MinMax  Function=max  Inputs=2  RndMeth=Simplest
  Multiport Switch1 : MultiPortSwitch  DataPortOrder=Zero-based contiguous  Inputs=2
  PT1 : Subsystem
  Product : Product  RndMeth=Simplest  SaturateOnIntegerOverflow=on
  RelationalOperator : RelationalOperator  Operator=<  OutDataTypeStr=boolean  RndMeth=Nearest
  Saturation Dynamic1 : Subsystem  mask(Saturation Dynamic){OutMin=[], OutMax=[], OutDataTypeStr=Inherit: Same as second input, OutputDataTypeScalingMode=Same as second input, OutDataType=fixdt(1, 16), OutScaling=2^-10, LockScale=off, RndMeth=Floor, DoSatur=off}
      mask prompts: OutMin "Simulink:masks:OutputMinimum_MP"; OutMax "Simulink:masks:OutputMaximum_MP"; OutDataTypeStr "Simulink:masks:OutputDataType_MP"; OutputDataTypeScalingMode "Simulink:masks:OutputDataTypeMode_MP"; OutDataType "Simulink:masks:OutputDataTypeegFixdt116Fixdtsingle_MP"; OutScaling "Simulink:masks:OutputScalingSlopeEg29OrSlopeBias_MP"; LockScale "Simulink:masks:LockOutputDataTypeAgainstFxpTools_MP"; RndMeth "Simulink:masks:IntegerRoundingMode_MP"; DoSatur "Simulink:masks:SaturateOnIntegerOverflow_MP"
      mask help: Simulink:masks:SaturationDynamic_MD
      mask init: same as Virtual_Exhaust_Aftertreatment_Controller_PRT/UCatCtrl/Urea_Dosing_Control/Saturation Dynamic
      mask Callback OutDataTypeStr: fixptdialog(gcbh)
      mask TypeOptions OutputDataTypeScalingMode: double | single | int8 | uint8 | int16 | uint16 | int32 | uint32 | Specify via dialog | Same as second input
      mask Callback OutputDataTypeScalingMode: fixptdialog(gcbh)
      mask Callback OutDataType: fixptdialog(gcbh)
      mask TypeOptions RndMeth: Simulink:masks:Ceiling | Simulink:masks:Convergent | Simulink:masks:Floor | Simulink:masks:Nearest | Simulink:masks:Round | Simulink:masks:Simplest | Simulink:masks:Zero
      mask Display: plot([0.15 0.85],[.5 .5],[.5 .5],[0.05 0.95],0.15+0.7*[0 .25 .75 1],0.05+0.9*[.25 .25 .75 .75]);
  Subtract : Sum  Inputs=+-  RndMeth=Simplest  SaturateOnIntegerOverflow=on
  TeQ : Subsystem
  UnitDelay1 : UnitDelay  InitialCondition=true  SampleTime=-1
      settings: AttributesFormatString=Init: %<X0>
  tUCatUsTEst : Outport
  wires:
  Subtract/1 -> Multiport Switch1/2
  tUCatUsT/1 -> Multiport Switch1/3, Subtract/1, RelationalOperator/1
  dwRdcAg/1 -> Add2/1
  dwPhChngWt/1 -> Add2/2
  dwUrea/1 -> Add2/3
  dwWtPreReac/1 -> Add2/4
  dwUreaReac/1 -> Add2/5
  dwWtPostReac/1 -> Add2/6
  dwNH3/1 -> Add2/7
  dwCO2/1 -> Add2/8
  Add2/1 -> Divide/1  "EvpMod_dwUCatUsTot_mp"
  dmEG/1 -> MinMax/1
  Product/1 -> Divide/2
  Divide/1 -> Saturation Dynamic1/2(u)
  Constant_1/1 -> MinMax/2
  MinMax/1 -> Product/1
  Constant_5/1 -> RelationalOperator/2
  Multiport Switch1/1 -> PT1/6(YReset), PT1/5(XReset), PT1/1(X)  "EvpMod_tUCatUsTUnFlt_mp"
  cpEG/1 -> Product/2
  PT1/1(Y) -> tUCatUsTEst/1
  Constant_4/1 -> PT1/2(K)
  Constant_6/1 -> TeQ/1(T)
  tiSampling/1 -> TeQ/2(dt)
  RelationalOperator/1 -> LogicalOperator1/1
  LogicalOperator/1 -> LogicalOperator1/2
  LogicalOperator1/1 -> Multiport Switch1/1
  Saturation Dynamic1/1(y) -> Subtract/2  "EvpMod_tDiffUCatUs_mp"
  Constant_2/1 -> Saturation Dynamic1/1(up)
  Constant_3/1 -> Saturation Dynamic1/3(lo)
  Constant_18/1 -> UnitDelay1/1
  UnitDelay1/1 -> PT1/4(Reset)
  LogicalOperator2/1 -> LogicalOperator/1  "FId_EvpModRls"
  Ground/1 -> LogicalOperator2/1
  TeQ/1(TeQ) -> PT1/3(TeQ)

== system Virtual_Exhaust_Aftertreatment_Controller_PRT/UCatCtrl/Urea_Dosing_Control/Feedback Control/Distribution Factor ==
  "ATS_rNOxUCatDs_ppm " : Inport
  ATS_rEstNOxUCatDs_ppm : Inport  Port=2
  ATS_rNOxUCatUs_ppm : Inport  Port=3
  Constant1 : Constant  Value=0  SampleTime=-1
  Constant3 : Constant  SampleTime=-1
  Constant_1 : Constant  Value=0.5  SampleTime=-1
  Distribution Factor Sat : Saturate  UpperLimit=1  LowerLimit=0
  Divide2 : Product  Inputs=*/
  Lookup_n-D_11 : Lookup_n-D  NumberOfTableDimensions=1  BreakpointsForDimension1=[0;10;20;50;100;200;500;1000]  BreakpointsForDimension2=[159.96 449.96]  Table=[0;1;2;5;10;20;50;100]  ExtrapMethod=Clip  UseLastTableValue=on  RndMeth=Simplest  InputSameDT=on
  MinMax : MinMax  Inputs=2
  MinMax1 : MinMax  Function=max  Inputs=2
  MinMax2 : MinMax  Function=max  Inputs=2
  Product1 : Product  RndMeth=Zero
  Subtract1 : Sum  Inputs=+-
  Subtract2 : Sum  Inputs=-+
  ATS_facDistbnCtl : Outport
  wires:
  "ATS_rNOxUCatDs_ppm "/1 -> Lookup_n-D_11/1
  ATS_rEstNOxUCatDs_ppm/1 -> MinMax/2
  Constant1/1 -> MinMax1/1
  Lookup_n-D_11/1 -> MinMax1/2
  MinMax1/1 -> Subtract2/1
  Constant3/1 -> MinMax2/2
  Subtract2/1 -> Divide2/1
  MinMax2/1 -> Divide2/2
  Divide2/1 -> Distribution Factor Sat/1
  Distribution Factor Sat/1 -> ATS_facDistbnCtl/1
  Product1/1 -> MinMax/1
  Constant_1/1 -> Product1/2
  ATS_rNOxUCatUs_ppm/1 -> Product1/1, Subtract1/1
  MinMax/1 -> Subtract1/2
  Subtract1/1 -> Subtract2/2, MinMax2/1

== system Virtual_Exhaust_Aftertreatment_Controller_PRT/UCatCtrl/Urea_Dosing_Control/Feedback Control/GOTO_ATS_facNOxCtl ==
  InXX : Inport
  GainXX : Subsystem
  tag scope: ATS_facNOxCtl=global
  wires:
  GainXX/1(Out) -> [ATS_facNOxCtl]  "ATS_facNOxCtl"
  InXX/1 -> GainXX/1(In)

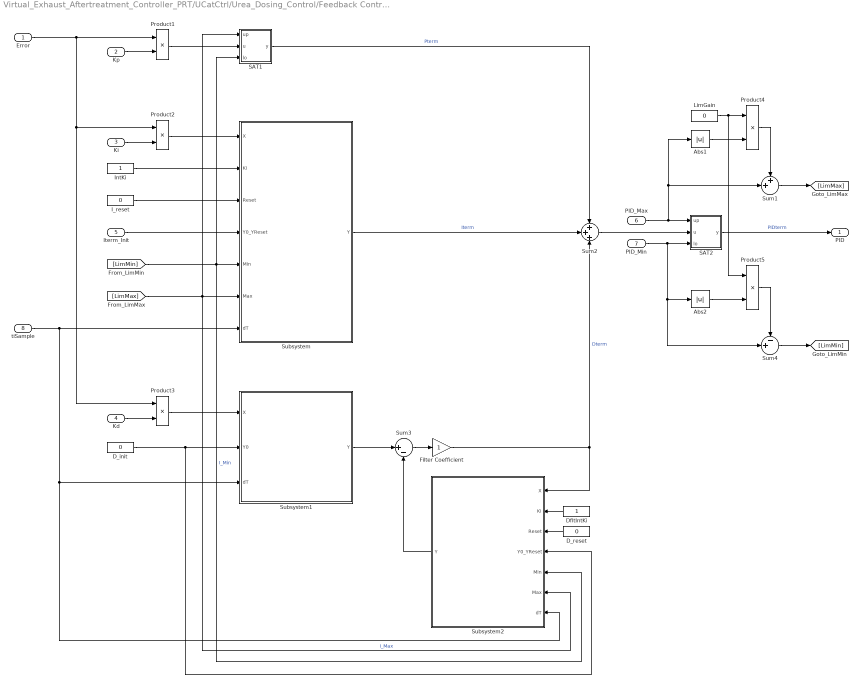
== system Virtual_Exhaust_Aftertreatment_Controller_PRT/UCatCtrl/Urea_Dosing_Control/Feedback Control/PIDctrl ==
  Error : Inport
  Kp : Inport  Port=2
  Ki : Inport  Port=3
  Kd : Inport  Port=4
  Iterm_Init : Inport  Port=5
  PID_Max : Inport  Port=6
  PID_Min : Inport  Port=7
  tiSample : Inport  Port=8
  Abs1 : Abs
  Abs2 : Abs
  D_init : Constant  Value=0  SampleTime=-1
  D_reset : Constant  Value=0  SampleTime=-1
  DfltIntKi : Constant  SampleTime=-1
  Filter Coefficient : Gain
  I_reset : Constant  Value=0  SampleTime=-1
  IntKi : Constant  SampleTime=-1
  LimGain : Constant  Value=0  SampleTime=-1
  Product{1..5} (5 alike) : Product  Inputs=**
  SAT1 : Subsystem  mask(Saturation Dynamic){OutMin=[], OutMax=[], OutDataTypeStr=Inherit: Same as second input, OutputDataTypeScalingMode=Same as second input, OutDataType=fixdt(1, 16), OutScaling=2^-10, LockScale=off, RndMeth=Floor, DoSatur=off}
      mask prompts: OutMin "Simulink:masks:OutputMinimum_MP"; OutMax "Simulink:masks:OutputMaximum_MP"; OutDataTypeStr "Simulink:masks:OutputDataType_MP"; OutputDataTypeScalingMode "Simulink:masks:OutputDataTypeMode_MP"; OutDataType "Simulink:masks:OutputDataTypeegFixdt116Fixdtsingle_MP"; OutScaling "Simulink:masks:OutputScalingSlopeEg29OrSlopeBias_MP"; LockScale "Simulink:masks:LockOutputDataTypeAgainstFxpTools_MP"; RndMeth "Simulink:masks:IntegerRoundingMode_MP"; DoSatur "Simulink:masks:SaturateOnIntegerOverflow_MP"
      mask help: Simulink:masks:SaturationDynamic_MD
      mask init: same as Virtual_Exhaust_Aftertreatment_Controller_PRT/UCatCtrl/Urea_Dosing_Control/Saturation Dynamic
      mask Callback OutDataTypeStr: fixptdialog(gcbh)
      mask TypeOptions OutputDataTypeScalingMode: double | single | int8 | uint8 | int16 | uint16 | int32 | uint32 | Specify via dialog | Same as second input
      mask Callback OutputDataTypeScalingMode: fixptdialog(gcbh)
      mask Callback OutDataType: fixptdialog(gcbh)
      mask TypeOptions RndMeth: Simulink:masks:Ceiling | Simulink:masks:Convergent | Simulink:masks:Floor | Simulink:masks:Nearest | Simulink:masks:Round | Simulink:masks:Simplest | Simulink:masks:Zero
      mask Display: plot([0.15 0.85],[.5 .5],[.5 .5],[0.05 0.95],0.15+0.7*[0 .25 .75 1],0.05+0.9*[.25 .25 .75 .75]);
  SAT2 : Subsystem  mask(Saturation Dynamic){OutMin=[], OutMax=[], OutDataTypeStr=Inherit: Same as second input, OutputDataTypeScalingMode=Same as second input, OutDataType=fixdt(1, 16), OutScaling=2^-10, LockScale=off, RndMeth=Floor, DoSatur=off}
      mask prompts: OutMin "Simulink:masks:OutputMinimum_MP"; OutMax "Simulink:masks:OutputMaximum_MP"; OutDataTypeStr "Simulink:masks:OutputDataType_MP"; OutputDataTypeScalingMode "Simulink:masks:OutputDataTypeMode_MP"; OutDataType "Simulink:masks:OutputDataTypeegFixdt116Fixdtsingle_MP"; OutScaling "Simulink:masks:OutputScalingSlopeEg29OrSlopeBias_MP"; LockScale "Simulink:masks:LockOutputDataTypeAgainstFxpTools_MP"; RndMeth "Simulink:masks:IntegerRoundingMode_MP"; DoSatur "Simulink:masks:SaturateOnIntegerOverflow_MP"
      mask help: Simulink:masks:SaturationDynamic_MD
      mask init: same as Virtual_Exhaust_Aftertreatment_Controller_PRT/UCatCtrl/Urea_Dosing_Control/Saturation Dynamic
      mask Callback OutDataTypeStr: fixptdialog(gcbh)
      mask TypeOptions OutputDataTypeScalingMode: double | single | int8 | uint8 | int16 | uint16 | int32 | uint32 | Specify via dialog | Same as second input
      mask Callback OutputDataTypeScalingMode: fixptdialog(gcbh)
      mask Callback OutDataType: fixptdialog(gcbh)
      mask TypeOptions RndMeth: Simulink:masks:Ceiling | Simulink:masks:Convergent | Simulink:masks:Floor | Simulink:masks:Nearest | Simulink:masks:Round | Simulink:masks:Simplest | Simulink:masks:Zero
      mask Display: plot([0.15 0.85],[.5 .5],[.5 .5],[0.05 0.95],0.15+0.7*[0 .25 .75 1],0.05+0.9*[.25 .25 .75 .75]);
  Subsystem : Subsystem
  Subsystem1 : Subsystem
  Subsystem2 : Subsystem
  Sum1 : Sum  Inputs=++|
  Sum2 : Sum  Inputs=+++
  Sum3 : Sum  Inputs=|+-
  Sum4 : Sum  Inputs=-+|
  PID : Outport
  wires:
  PID_Max/1 -> SAT2/1(up), Sum1/2, Abs1/1
  Ki/1 -> Product2/2
  Kp/1 -> Product1/2
  Kd/1 -> Product3/2
  SAT1/1(y) -> Sum2/1  "Pterm"
  SAT2/1(y) -> PID/1  "PIDterm"
  IntKi/1 -> Subsystem/2(Ki)
  Subsystem/1(Y) -> Sum2/2  "Iterm"
  I_reset/1 -> Subsystem/3(Reset)
  [LimMin] -> Subsystem2/5(Min), Subsystem/5(Min), SAT1/3(lo)  "I_Min"
  tiSample/1 -> Subsystem/7(dT), Subsystem1/3(dT), Subsystem2/7(dT)
  [LimMax] -> Subsystem2/6(Max), Subsystem/6(Max), SAT1/1(up)  "I_Max"
  Error/1 -> Product1/1, Product3/1, Product2/1
  Sum2/1 -> SAT2/2(u)
  Iterm_Init/1 -> Subsystem/4(Y0_YReset)
  D_init/1 -> Subsystem1/2(Y0), Subsystem2/4(Y0_YReset)
  Filter Coefficient/1 -> Subsystem2/1(X), Sum2/3  "Dterm"
  Sum3/1 -> Filter Coefficient/1
  Subsystem1/1(Y) -> Sum3/1
  D_reset/1 -> Subsystem2/3(Reset)
  DfltIntKi/1 -> Subsystem2/2(Ki)
  Subsystem2/1(Y) -> Sum3/2
  Product1/1 -> SAT1/2(u)
  Product2/1 -> Subsystem/1(X)
  Product3/1 -> Subsystem1/1(X)
  Abs1/1 -> Product4/2
  Product4/1 -> Sum1/1
  Sum1/1 -> [LimMax]
  PID_Min/1 -> Sum4/2, Abs2/1, SAT2/3(lo)
  Abs2/1 -> Product5/2
  LimGain/1 -> Product5/1, Product4/1
  Product5/1 -> Sum4/1
  Sum4/1 -> [LimMin]

== system Virtual_Exhaust_Aftertreatment_Controller_PRT/UCatCtrl/Urea_Dosing_Control/GOTO_ATS_facQtyAdap/GainXX ==
  In : Inport
  Out : Outport
  wires:
  In/1 -> Out/1

== system Virtual_Exhaust_Aftertreatment_Controller_PRT/UCatCtrl/Urea_Dosing_Control/GOTO_ATS_mNH3LdNom/GainXX ==
  In : Inport
  Out : Outport
  wires:
  In/1 -> Out/1

== system Virtual_Exhaust_Aftertreatment_Controller_PRT/UCatCtrl/Urea_Dosing_Control/GOTO_ATS_mNH3LoadUCatRst/GainXX ==
  In : Inport
  Out : Outport
  wires:
  In/1 -> Out/1

== system Virtual_Exhaust_Aftertreatment_Controller_PRT/UCatCtrl/Urea_Dosing_Control/GOTO_ATS_mflNH3Cnv_mgps/GainXX ==
  In : Inport
  Out : Outport
  wires:
  In/1 -> Out/1

== system Virtual_Exhaust_Aftertreatment_Controller_PRT/UCatCtrl/Urea_Dosing_Control/GOTO_ATS_mflNH3CurrEfc_mgps/GainXX ==
  In : Inport
  Out : Outport
  wires:
  In/1 -> Out/1

== system Virtual_Exhaust_Aftertreatment_Controller_PRT/UCatCtrl/Urea_Dosing_Control/GOTO_ATS_mflNH3DpstLmt_mgps/GainXX ==
  In : Inport
  Out : Outport
  wires:
  In/1 -> Out/1

== system Virtual_Exhaust_Aftertreatment_Controller_PRT/UCatCtrl/Urea_Dosing_Control/GOTO_ATS_mflNH3MetAdapDes_mgps/GainXX ==
  In : Inport
  Out : Outport
  wires:
  In/1 -> Out/1

== system Virtual_Exhaust_Aftertreatment_Controller_PRT/UCatCtrl/Urea_Dosing_Control/GOTO_ATS_mflNH3PreCtl_mgps/GainXX ==
  In : Inport
  Out : Outport
  wires:
  In/1 -> Out/1

== system Virtual_Exhaust_Aftertreatment_Controller_PRT/UCatCtrl/Urea_Dosing_Control/GOTO_ATS_mflNH3_mgps/GainXX ==
  In : Inport
  Out : Outport
  wires:
  In/1 -> Out/1

== system Virtual_Exhaust_Aftertreatment_Controller_PRT/UCatCtrl/Urea_Dosing_Control/GOTO_ATS_mflNOxUs_mgps/GainXX ==
  In : Inport
  Out : Outport
  wires:
  In/1 -> Out/1

== system Virtual_Exhaust_Aftertreatment_Controller_PRT/UCatCtrl/Urea_Dosing_Control/GOTO_ATS_stNH3LoadUCatRst/GainXX ==
  In : Inport
  Out : Outport
  wires:
  In/1 -> Out/1

== system Virtual_Exhaust_Aftertreatment_Controller_PRT/UCatCtrl/Urea_Dosing_Control/GOTO_ATS_stUDosing/GainXX ==
  In : Inport
  Out : Outport
  wires:
  In/1 -> Out/1

== system Virtual_Exhaust_Aftertreatment_Controller_PRT/UCatCtrl/Urea_Dosing_Control/GOTO_EvpMod_tUCatUsT/GainXX ==
  In : Inport
  Out : Outport
  wires:
  In/1 -> Out/1

== system Virtual_Exhaust_Aftertreatment_Controller_PRT/UCatCtrl/Urea_Dosing_Control/Load Governor/Nominal Load ==
  ATS_volUCat : Inport
  ATS_tUCatAvrg : Inport  Port=2
  ATS_mflEG : Inport  Port=3
  ATS_facEffUCatAge : Inport  Port=4
  Interpolation Using Prelookup : Interpolation_n-D  NumberOfTableDimensions=1  TableSource=Input port  Table=|  ExtrapMethod=Clip  ValidIndexMayReachLast=on
      | [    0.2790    0.2970    0.3080    0.3220    0.3510    0.4240    0.5640    0.6550    0.8190    1.0000    1.0000    1.0000
      |     0.3260    0.3430    0.3540    0.3670    0.3960    0.4660    0.6010    0.6900    0.8440    1.0000    1.0000    1.0000
      |     0.3730    0.3890    0.4000    0.4130    0.4400    0.5080    0.6380    0.7230    0.8680    1.0000    1.0000    1.0000
      |     0.4320    0.4480    0.4580    0.4700    0.4960    0.5600    0.6830    0.7640    0.8970    1.0000    1.0000    1.0000
      |     0.4920    0.5070    0.5160    0.5270    0.5520    0.6120    0.7260    0.8020    0.9220    1.0000    1.0000    1.0000
      |     0.5510    0.5650    0.5730    0.5840    0.6070    0.6620    0.7680    0.8370    0.9410    1.0000    1.0000    1.0000
      |     0.6070    0.6200    0.6280    0.6380    0.6600    0.7130    0.8130    0.8750    0.9580    1.0000    1.0000    1.0000
      |     0.6580    0.6710    0.6790    0.6890    0.7110    0.7630    0.8600    0.9130    0.9730    1.0000    1.0000    1.0000
      |     0.7030    0.7170    0.7250    0.7360    0.7580    0.8130    0.9110    0.9540    0.9900    1.0000    1.0000    1.0000
      |     0.7620    0.7790    0.7900    0.8030    0.8300    0.8980    1.0000    1.0000    1.0000    1.0000    1.0000    1.0000
      |     0.7840    0.7980    0.8060    0.8160    0.8370    0.8910    0.9920    1.0000    1.0000    1.0000    1.0000    1.0000
      |     0.7800    0.8780    0.8820    0.8860    0.8950    0.9180    0.9620    1.0000    1.0000    1.0000    1.0000    1.0000
      | ]
      settings: InputPortMap=u0,u1,p2
  Interpolation_n-D_1 : Interpolation_n-D  Table=[0.885 0.845 0.814 0.674 0.631 0.547 0.458 0.379 0.242 0.131 0.091 0.025;0.885 0.845 0.814 0.674 0.631 0.547 0.458 0.379 0.242 0.131 0.091 0.025;0.885 0.845 0.814 0.674 0.631 0.547 0.458 0.379 0.242 0.131 0.091 0.025;0.885 0.845 0.814 0.674 0.631 0.547 0.458 0.379 0.242 0.131 0.091 0.025;0.885 0.845 0.814 0.674 0.631 0.547 0.458 0.379 0.242 0.131 0.091 0.025;0.885 0.845 0.814 0.674 0.631 0.547 0.458 0.379 0.242 0.131 0.091 0.025;0.885 0.845 0.814 0.674 0.631 0.547 0.458 0.379 0.242 0.131 0.091 0.025;0.885 0.845 0.814 0.674 0.631 0.547 0.458 0.379 0.242 0.131 0.091 0.025;0.885 0.845 0.814 0.674 0.631 0.547 0.458 0.379 0.242 0.131 0.091 0.025;0.885 0.845 0.814 0.674 0.631 0.547 0.458 0.379 0.242 0.131 0.091 0.025;0.885 0.845 0.814 0.674 0.631 0.547 0.458 0.379 0.242 0.131 0.091 0.025;0.885 0.845 0.814 0.674 0.631 0.547 0.458 0.379 0.242 0.131 0.091 0.025]  ExtrapMethod=Clip
  Interpolation_n-D_2 : Interpolation_n-D  Table=[0.893 0.852 0.82 0.675 0.632 0.549 0.46 0.381 0.243 0.132 0.092 0.025;0.893 0.852 0.82 0.675 0.632 0.549 0.46 0.381 0.243 0.132 0.092 0.025;0.893 0.852 0.82 0.675 0.632 0.549 0.46 0.381 0.243 0.132 0.092 0.025;0.893 0.852 0.82 0.675 0.632 0.549 0.46 0.381 0.243 0.132 0.092 0.025;0.893 0.852 0.82 0.675 0.632 0.549 0.46 0.381 0.243 0.132 0.092 0.025;0.893 0.852 0.82 0.675 0.632 0.549 0.46 0.381 0.243 0.132 0.092 0.025;0.893 0.852 0.82 0.675 0.632 0.549 0.46 0.381 0.243 0.132 0.092 0.025;0.893 0.852 0.82 0.675 0.632 0.549 0.46 0.381 0.243 0.132 0.092 0.025;0.893 0.852 0.82 0.675 0.632 0.549 0.46 0.381 0.243 0.132 0.092 0.025;0.893 0.852 0.82 0.675 0.632 0.549 0.46 0.381 0.243 0.132 0.092 0.025;0.893 0.852 0.82 0.675 0.632 0.549 0.46 0.381 0.243 0.132 0.092 0.025;0.893 0.852 0.82 0.675 0.632 0.549 0.46 0.381 0.243 0.132 0.092 0.025]  ExtrapMethod=Clip
  Lookup_n-D_3 : Lookup_n-D  BreakpointsForDimension1=[0;0.143;0.286;0.429;0.571;0.714;0.857;1]  BreakpointsForDimension2=[159.96 179.96 199.96 224.96 249.96 274.96 299.96 324.96 349.96 374.96 399.96 424.96]  Table=[0 0 0 0 0 0 0 0 0 0 0 0;0.143 0.143 0.143 0.143 0.143 0.143 0.143 0.143 0.143 0.143 0.143 0.143;0.286 0.286 0.286 0.286 0.286 0.286 0.286 0.286 0.286 0.286 0.286 0.286;0.429 0.429 0.429 0.429 0.429 0.429 0.429 0.429 0.429 0.429 0.429 0.429;0.571 0.571 0.571 0.571 0.571 0.571 0.571 0.571 0.571 0.571 0.571 0.571;0.714 0.714 0.714 0.714 0.714 0.714 0.714 0.714 0.714 0.714 0.714 0.714;0.857 0.857 0.857 0.857 0.857 0.857 0.857 0.857 0.857 0.857 0.857 0.857;1 1 1 1 1 1 1 1 1 1 1 1]  ExtrapMethod=Clip  UseLastTableValue=on  RndMeth=Simplest  InputSameDT=on
  Mux1 : Mux  Inputs=2
  PreLookup_1 : PreLookup  BreakpointsData=[0;50;100;150;200;300;400;600;800;1000;1200;1400]  ExtrapMethod=Linear
  PreLookup_2 : PreLookup  BreakpointsData=[179.96;199.96;224.96;249.96;274.96;299.96;324.96;349.96;374.96;399.96;424.96;499.96]  ExtrapMethod=Linear
  Prelookup : PreLookup  BreakpointsData=|  UseLastBreakpoint=on
      | [  0 1.0
      | ]
  Product2 : Product  RndMeth=Zero
  ATS_mNH3LdNom_g : Outport
  wires:
  ATS_mflEG/1 -> PreLookup_1/1
  ATS_tUCatAvrg/1 -> Lookup_n-D_3/2, PreLookup_2/1
  Interpolation_n-D_1/1 -> Mux1/1
  Interpolation_n-D_2/1 -> Mux1/2
  Mux1/1 -> Interpolation Using Prelookup/3
  Lookup_n-D_3/1 -> Prelookup/1
  Interpolation Using Prelookup/1 -> Product2/1
  PreLookup_2/1 -> Interpolation_n-D_1/3, Interpolation_n-D_2/3
  PreLookup_2/2 -> Interpolation_n-D_1/4, Interpolation_n-D_2/4
  Prelookup/1 -> Interpolation Using Prelookup/1
  Prelookup/2 -> Interpolation Using Prelookup/2
  PreLookup_1/2 -> Interpolation_n-D_2/2, Interpolation_n-D_1/2
  PreLookup_1/1 -> Interpolation_n-D_2/1, Interpolation_n-D_1/1
  ATS_volUCat/1 -> Product2/2
  Product2/1 -> ATS_mNH3LdNom_g/1
  ATS_facEffUCatAge/1 -> Lookup_n-D_3/1
